simulink library "lib_TCML"  (R2015a)
settings: Solver=ode45  StartTime=0.0  StopTime=10.0  RelTol=1e-3
libraries: simulink x5
(part 4 of 7)

== system lib_TCML/Dynamic Tip Clearance/Case Deformation/Deformation1 ==
  Average Temperature(R) : Inport
  Memory : Memory  X0=mean(T0_Case_M)
  Memory3 : Memory  X0=Ri_Case_M
  Thermal Expansion 1D Elastic : Subsystem  mask(TSAT: Thermal Expansion Library Block){TempDependence_M=on, alpha_M=alpha_Case_M, T_data_M=Talpha_Case_Data_M, alpha_data_M=alpha_Case_Data_M, BN_M=double(gcb)}
      mask prompts: TempDependence_M "TempDependence_M - Temperature dependence of the thermal expansion coefficient (unchecked - constant, checked - temperature dependent)"; alpha_M "alpha_M - Constant thermal expansion coefficient"; T_data_M "T_data_M - Temperature array (nx1)"; alpha_data_M "alpha_data_M - Thermal expansion coefficient array (nx1)"; BN_M "Block Name"
      mask help:
      | This function calculates the length or radius of a structure that has expanded or contracted due to thermal expansion. The block accepts the previous/reference length (Lo), previous/reference temperature (To), and current temperature (Tf) as its inputs. The user has the option to specify a constant thermal expansion coefficient or to incorporate temperature dependence by providing data that correlates the thermal expansion coefficient with temperature.
      |
      | This block is capable of accepting various units but it is important that the units be consistent across all inputs and parameters. For details on this block, see the block help menu.
      mask init:
      | %set default parameters if they are not being used
      | if TempDependence_M == 0
      |     T_data_M = [0 5000];
      |     alpha_data_M = [10e-6 10e-6];
      | elseif TempDependence_M == 1
      |     alpha_M = 10e-6;
      | end
      mask Help: web(which('Deformation_TSAT_ThermExp1DElastic.html'),'-helpbrowser')
      mask Callback TempDependence_M:
      | MSK_SEC_Enables_TSAT('TempDependence_M',2,'dis')
      | MSK_SEC_Enables_TSAT('TempDependence_M',[3 4],'en')
  Case Radius (ft) : Outport
  wires:
  Thermal Expansion 1D Elastic/1(Current Length [L]) -> Memory3/1, Case Radius (ft)/1
  Average Temperature(R)/1 -> Memory/1, Thermal Expansion 1D Elastic/3(Current Temperature [Tf])
  Memory/1 -> Thermal Expansion 1D Elastic/2(Previous/Reference Temperature [To])
  Memory3/1 -> Thermal Expansion 1D Elastic/1(Previous/Reference Length [Lo])

== system lib_TCML/Dynamic Tip Clearance/Case Deformation/Thermal Properties ==
  Temperature [T] : Inport
  Density (Abradable Material) : Constant  Value=rho_Case_M * ones(1,n_Case_M)  SampleTime=dt_Case_M
  Heat Capacity vs. Temperature (Abradable Material) : Lookup_n-D  NumberOfTableDimensions=1  BreakpointsForDimension1=TCp_Case_Data_M  Table=Cp_Case_Data_M  InternalRulePriority=Speed  RndMeth=Simplest  InputSameDT=on
  Is k of temperature dependent : Constant  Value=k_TempDependence_Case_M  SampleTime=dt_Case_M
  Is k of temperature dependent1 : Constant  Value=Cp_TempDependence_Case_M  SampleTime=dt_Case_M
  Switch1 : Switch  Criteria=u2 > Threshold
  Switch2 : Switch  Criteria=u2 > Threshold
  Thermal Conductivity (Abradable Material) : Constant  Value=k_Case_M * ones(1,n_Case_M)  SampleTime=dt_Case_M
  Thermal Conductivity (Abradable Material)1 : Constant  Value=Cp_Case_M * ones(1,n_Case_M)  SampleTime=dt_Case_M
  Thermal Conductivity vs. Temperature (Abradable Material) : Lookup_n-D  NumberOfTableDimensions=1  BreakpointsForDimension1=Tk_Case_Data_M  Table=k_Case_Data_M  InternalRulePriority=Speed  RndMeth=Simplest  InputSameDT=on
  Thermal Conductivity [k] : Outport
  Heat Capacity [Cp] : Outport  Port=2
  Density [rho] : Outport  Port=3
  wires:
  Switch1/1 -> Heat Capacity [Cp]/1
  Is k of temperature dependent1/1 -> Switch1/2
  Thermal Conductivity (Abradable Material)1/1 -> Switch1/3
  Is k of temperature dependent/1 -> Switch2/2
  Thermal Conductivity (Abradable Material)/1 -> Switch2/3
  Thermal Conductivity vs. Temperature (Abradable Material)/1 -> Switch2/1
  Switch2/1 -> Thermal Conductivity [k]/1
  Density (Abradable Material)/1 -> Density [rho]/1
  Temperature [T]/1 -> Thermal Conductivity vs. Temperature (Abradable Material)/1, Heat Capacity vs. Temperature (Abradable Material)/1
  Heat Capacity vs. Temperature (Abradable Material)/1 -> Switch1/1

== system lib_TCML/Dynamic Tip Clearance/Case Deformation/While Iterator Subsystem ==
  Tin (R)1 : Inport
  hin (Btu/(sec-ft^2-R))1 : Inport  Port=2
  Tout (R)1 : Inport  Port=3
  hout (Btu/(sec-ft^2-R))1 : Inport  Port=4
  Abs2 : Abs
  Add2 : Sum  Inputs=-+
  Compare To Constant2 : simulink/Logic and Bit Operations/Compare To Constant  relop=>=  const=0.1  OutDataTypeStr=boolean
  Is k of temperature dependent1 : Constant  Value=k_TempDependence_Case_M  SampleTime=-1
  MATLAB Function1 : MATLAB Function  TreatAsAtomicUnit=on
  Memory5 : Memory  X0=mean(T0_Case_M)  InheritSampleTime=on
  Memory6 : Memory  X0=mean(T0_Case_M)  InheritSampleTime=on
  Switch : Switch  Criteria=u2 > Threshold
  Thermal Conductivity (Abradable Material)1 : Constant  Value=k_Case_M  SampleTime=-1
  Thermal Conductivity vs. Temperature : Lookup_n-D  NumberOfTableDimensions=1  BreakpointsForDimension1=Tk_Case_Data_M  Table=k_Case_Data_M  InternalRulePriority=Speed  RndMeth=Simplest  InputSameDT=on
  While Iterator : WhileIterator  MaxIters=1000  WhileBlockType=do-while
  Width of Rotor : Constant  Value=W_Case_M  SampleTime=-1
  Tavg (R) : Outport
  wires:
  Thermal Conductivity vs. Temperature/1 -> Switch/1
  Is k of temperature dependent1/1 -> Switch/2
  Thermal Conductivity (Abradable Material)1/1 -> Switch/3
  Compare To Constant2/1 -> While Iterator/1
  Abs2/1 -> Compare To Constant2/1
  Add2/1 -> Abs2/1
  Memory5/1 -> Add2/1
  Memory6/1 -> Thermal Conductivity vs. Temperature/1
  MATLAB Function1/1(Tavg) -> Memory5/1, Memory6/1, Add2/2, Tavg (R)/1
  Switch/1 -> MATLAB Function1/1(k)
  hout (Btu/(sec-ft^2-R))1/1 -> MATLAB Function1/6(hout)
  Tout (R)1/1 -> MATLAB Function1/5(Tout)
  hin (Btu/(sec-ft^2-R))1/1 -> MATLAB Function1/4(hin)
  Tin (R)1/1 -> MATLAB Function1/3(Tin)
  Width of Rotor/1 -> MATLAB Function1/2(W)

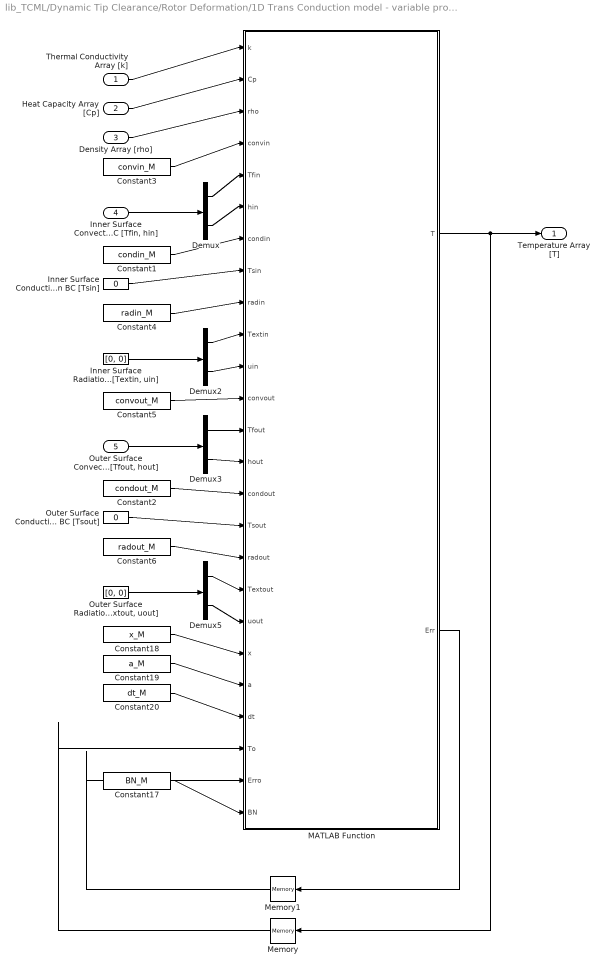
== system lib_TCML/Dynamic Tip Clearance/Rotor Deformation/1D Trans Conduction model - variable props & general BCs ==
  Thermal Conductivity Array [k] : Inport
  Heat Capacity Array [Cp] : Inport  Port=2
  Density Array [rho] : Inport  Port=3
  "Inner Surface Convection BC [Tfin, hin]" : Inport  Port=4
  "Outer Surface Convection BC [Tfout, hout]" : Inport  Port=5
  Constant1 : Constant  Value=condin_M
  Constant17 : Constant  Value=BN_M
  Constant18 : Constant  Value=x_M
  Constant19 : Constant  Value=a_M
  Constant2 : Constant  Value=condout_M
  Constant20 : Constant  Value=dt_M
  Constant3 : Constant  Value=convin_M
  Constant4 : Constant  Value=radin_M
  Constant5 : Constant  Value=convout_M
  Constant6 : Constant  Value=radout_M
  Demux{,2..3,5} (4 alike) : Demux  Outputs=[1 1]
  Inner Surface Conduction BC [Tsin] : Constant  Value=0
  "Inner Surface Radiation BC [Textin, uin]" : Constant  Value=[0, 0]
  MATLAB Function : MATLAB Function  TreatAsAtomicUnit=on  SystemSampleTime=dt_M
  Memory : Memory  X0=T0_M  InheritSampleTime=on
  Memory1 : Memory  X0=zeros(1,37)  InheritSampleTime=on
  Outer Surface Conduction BC [Tsout] : Constant  Value=0
  "Outer Surface Radiation BC [Textout, uout]" : Constant  Value=[0, 0]
  Temperature Array [T] : Outport
  wires:
  "Outer Surface Radiation BC [Textout, uout]"/1 -> Demux5/1
  Demux5/2 -> MATLAB Function/19(uout)
  Demux5/1 -> MATLAB Function/18(Textout)
  Outer Surface Conduction BC [Tsout]/1 -> MATLAB Function/16(Tsout)
  Demux3/2 -> MATLAB Function/14(hout)
  Demux3/1 -> MATLAB Function/13(Tfout)
  "Outer Surface Convection BC [Tfout, hout]"/1 -> Demux3/1
  Demux2/2 -> MATLAB Function/11(uin)
  Demux2/1 -> MATLAB Function/10(Textin)
  "Inner Surface Radiation BC [Textin, uin]"/1 -> Demux2/1
  Inner Surface Conduction BC [Tsin]/1 -> MATLAB Function/8(Tsin)
  Demux/2 -> MATLAB Function/6(hin)
  Demux/1 -> MATLAB Function/5(Tfin)
  "Inner Surface Convection BC [Tfin, hin]"/1 -> Demux/1
  Constant6/1 -> MATLAB Function/17(radout)
  Constant5/1 -> MATLAB Function/12(convout)
  Constant4/1 -> MATLAB Function/9(radin)
  Constant3/1 -> MATLAB Function/4(convin)
  Constant2/1 -> MATLAB Function/15(condout)
  Constant1/1 -> MATLAB Function/7(condin)
  MATLAB Function/2(Err) -> Memory1/1
  Memory/1 -> MATLAB Function/23(To)
  MATLAB Function/1(T) -> Temperature Array [T]/1, Memory/1
  Constant20/1 -> MATLAB Function/22(dt)
  Constant19/1 -> MATLAB Function/21(a)
  Constant18/1 -> MATLAB Function/20(x)
  Density Array [rho]/1 -> MATLAB Function/3(rho)
  Heat Capacity Array [Cp]/1 -> MATLAB Function/2(Cp)
  Thermal Conductivity Array [k]/1 -> MATLAB Function/1(k)
  Memory1/1 -> MATLAB Function/24(Erro)
  Constant17/1 -> MATLAB Function/25(BN)

== system lib_TCML/Dynamic Tip Clearance/Rotor Deformation/Convective Heat Transfer Coefficient on Back Surface ==
  Mass Flow Rate [W] : Inport
  Fluid Temperature [T] : Inport  Port=2
  2-D Lookup Table : Lookup_n-D  BreakpointsForDimension1=Wc_Rotor_Back_Data_M  BreakpointsForDimension2=Tc_Rotor_Back_Data_M  Table=h_Rotor_Back_Data_M  InternalRulePriority=Speed  RndMeth=Simplest  InputSameDT=on
  Constant : Constant  Value=0.8  SampleTime=dt_Rotor_M
  Constant1 : Constant  Value=0.23  SampleTime=dt_Rotor_M
  Convective Heat Transfer Coefficient : Constant  Value=h_Rotor_Back_M  SampleTime=dt_Rotor_M
  Gain : Gain  Gain=hcoeff_Rotor_Back_M
  Gain1 : Gain  Gain=1/Wdes_Rotor_Back_M
  Gain2 : Gain  Gain=1/Tdes_Rotor_Back_M
  Math Function : Math  Operator=pow  SaturateOnIntegerOverflow=on
  Math Function1 : Math  Operator=pow  SaturateOnIntegerOverflow=on
  Multiport Switch : MultiPortSwitch
  Product : Product
  Which Convective Heat Transfer Coefficient Model? : Constant  Value=ConvHeatXCoeffMdl_Rotor_Back_I  SampleTime=dt_Rotor_M
  Convective Heat Transfer Coefficient [h] : Outport
  wires:
  Multiport Switch/1 -> Convective Heat Transfer Coefficient [h]/1
  2-D Lookup Table/1 -> Multiport Switch/4
  Constant/1 -> Math Function/2
  Which Convective Heat Transfer Coefficient Model?/1 -> Multiport Switch/1
  Gain/1 -> Multiport Switch/3
  Mass Flow Rate [W]/1 -> Gain1/1
  Convective Heat Transfer Coefficient/1 -> Multiport Switch/2
  Gain1/1 -> 2-D Lookup Table/2, Math Function/1
  Constant1/1 -> Math Function1/2
  Fluid Temperature [T]/1 -> Gain2/1
  Gain2/1 -> 2-D Lookup Table/1, Math Function1/1
  Math Function/1 -> Product/1
  Math Function1/1 -> Product/2
  Product/1 -> Gain/1

== system lib_TCML/Dynamic Tip Clearance/Rotor Deformation/Convective Heat Transfer Coefficient on Front Surface ==
  Mass Flow Rate [W] : Inport
  Fluid Temperature [T] : Inport  Port=2
  2-D Lookup Table : Lookup_n-D  BreakpointsForDimension1=Wc_Rotor_Front_Data_M  BreakpointsForDimension2=Tc_Rotor_Front_Data_M  Table=h_Rotor_Front_Data_M  InternalRulePriority=Speed  RndMeth=Simplest  InputSameDT=on
  Constant : Constant  Value=0.8  SampleTime=dt_Rotor_M
  Constant1 : Constant  Value=0.23  SampleTime=dt_Rotor_M
  Convective Heat Transfer Coefficient : Constant  Value=h_Rotor_Front_M  SampleTime=dt_Rotor_M
  Gain : Gain  Gain=hcoeff_Rotor_Front_M
  Gain1 : Gain  Gain=1/Wdes_Rotor_Front_M
  Gain2 : Gain  Gain=1/Tdes_Rotor_Front_M
  Math Function : Math  Operator=pow  SaturateOnIntegerOverflow=on
  Math Function1 : Math  Operator=pow  SaturateOnIntegerOverflow=on
  Multiport Switch : MultiPortSwitch
  Product : Product
  Which Convective Heat Transfer Coefficient Model? : Constant  Value=ConvHeatXCoeffMdl_Rotor_Front_I  SampleTime=dt_Rotor_M
  Convective Heat Transfer Coefficient [h] : Outport
  wires:
  Product/1 -> Gain/1
  Math Function1/1 -> Product/2
  Math Function/1 -> Product/1
  Gain2/1 -> Math Function1/1, 2-D Lookup Table/1
  Fluid Temperature [T]/1 -> Gain2/1
  Constant1/1 -> Math Function1/2
  Gain1/1 -> Math Function/1, 2-D Lookup Table/2
  Convective Heat Transfer Coefficient/1 -> Multiport Switch/2
  Mass Flow Rate [W]/1 -> Gain1/1
  Gain/1 -> Multiport Switch/3
  Which Convective Heat Transfer Coefficient Model?/1 -> Multiport Switch/1
  Constant/1 -> Math Function/2
  2-D Lookup Table/1 -> Multiport Switch/4
  Multiport Switch/1 -> Convective Heat Transfer Coefficient [h]/1

== system lib_TCML/Dynamic Tip Clearance/Rotor Deformation/Deformation ==
  Average Temperature (R) : Inport
  Shaft Speed (rpm) : Inport  Port=2
  Deformation Due To Centrifugal Forces : Subsystem
  Deformation Due To Thermal Expansion : Subsystem
  Subtract : Sum
  Rotor Outer Radius (ft) : Outport
  Unstrained Rotor Outer Radius (ft) : Outport  Port=2
  wires:
  Average Temperature (R)/1 -> Deformation Due To Centrifugal Forces/2(Average Temperature), Deformation Due To Thermal Expansion/1(Average Rotor Temperature)
  Subtract/1 -> Rotor Outer Radius (ft)/1
  Shaft Speed (rpm)/1 -> Deformation Due To Centrifugal Forces/1(Shaft Speed [N] (rpm))
  Deformation Due To Centrifugal Forces/1(Rotor Radius) -> Subtract/1
  Deformation Due To Thermal Expansion/1(Rotor Radius after Thermal Expansion) -> Unstrained Rotor Outer Radius (ft)/1, Subtract/2, Deformation Due To Centrifugal Forces/3(Rotor Radius After Thermal Expansion)

== system lib_TCML/Dynamic Tip Clearance/Rotor Deformation/Deformation1 ==
  Average Temperature (R) : Inport
  Shaft Speed (rpm) : Inport  Port=2
  Deformation Due To Centrifugal Forces : Subsystem
  Deformation Due To Thermal Expansion : Subsystem
  Subtract : Sum
  Rotor Outer Radius (ft) : Outport
  wires:
  Deformation Due To Thermal Expansion/1(Rotor Radius after Thermal Expansion) -> Deformation Due To Centrifugal Forces/3(Rotor Radius After Thermal Expansion), Subtract/2
  Deformation Due To Centrifugal Forces/1(Rotor Radius) -> Subtract/1
  Shaft Speed (rpm)/1 -> Deformation Due To Centrifugal Forces/1(Shaft Speed [N] (rpm))
  Subtract/1 -> Rotor Outer Radius (ft)/1
  Average Temperature (R)/1 -> Deformation Due To Thermal Expansion/1(Average Rotor Temperature), Deformation Due To Centrifugal Forces/2(Average Temperature)

== system lib_TCML/Dynamic Tip Clearance/Rotor Deformation/Thermal Properties ==
  Temperature [T] : Inport
  Density (Super Alloy) : Constant  Value=rho_Rotor_M * ones(1,n_Rotor_M)  SampleTime=dt_Rotor_M
  Heat Capacity vs. Temperature : Lookup_n-D  NumberOfTableDimensions=1  BreakpointsForDimension1=TCp_Rotor_Data_M  Table=Cp_Rotor_Data_M  InternalRulePriority=Speed  RndMeth=Simplest  InputSameDT=on
  Is k of temperature dependent : Constant  Value=k_TempDependence_Rotor_M  SampleTime=dt_Rotor_M
  Is k of temperature dependent1 : Constant  Value=Cp_TempDependence_Rotor_M  SampleTime=dt_Rotor_M
  Switch : Switch  Criteria=u2 > Threshold
  Switch1 : Switch  Criteria=u2 > Threshold
  Thermal Conductivity (Abradable Material) : Constant  Value=k_Rotor_M * ones(1,n_Rotor_M)  SampleTime=dt_Rotor_M
  Thermal Conductivity (Super Alloy)1 : Constant  Value=Cp_Rotor_M * ones(1,n_Rotor_M)  SampleTime=dt_Rotor_M
  Thermal Conductivity vs. Temperature : Lookup_n-D  NumberOfTableDimensions=1  BreakpointsForDimension1=Tk_Rotor_Data_M  Table=k_Rotor_Data_M  InternalRulePriority=Speed  RndMeth=Simplest  InputSameDT=on
  Thermal Conductivity [k] : Outport
  Heat Capacity [Cp] : Outport  Port=2
  Density [rho] : Outport  Port=3
  wires:
  Temperature [T]/1 -> Heat Capacity vs. Temperature/1, Thermal Conductivity vs. Temperature/1
  Thermal Conductivity (Super Alloy)1/1 -> Switch1/3
  Thermal Conductivity vs. Temperature/1 -> Switch/1
  Switch/1 -> Thermal Conductivity [k]/1
  Is k of temperature dependent/1 -> Switch/2
  Heat Capacity vs. Temperature/1 -> Switch1/1
  Switch1/1 -> Heat Capacity [Cp]/1
  Is k of temperature dependent1/1 -> Switch1/2
  Thermal Conductivity (Abradable Material)/1 -> Switch/3
  Density (Super Alloy)/1 -> Density [rho]/1

== system lib_TCML/Dynamic Tip Clearance/Rotor Deformation/While Iterator Subsystem ==
  Tin (R) : Inport
  hin (Btu/(sec-ft^2-R)) : Inport  Port=2
  Tout (R) : Inport  Port=3
  hout (Btu/(sec-ft^2-R)) : Inport  Port=4
  Abs : Abs
  Add : Sum  Inputs=-+
  Compare To Constant : simulink/Logic and Bit Operations/Compare To Constant  relop=>=  const=0.1  OutDataTypeStr=boolean
  Is k of temperature dependent : Constant  Value=k_TempDependence_Rotor_M  SampleTime=-1
  MATLAB Function1 : MATLAB Function  TreatAsAtomicUnit=on
  Memory1 : Memory  X0=mean(T0_Rotor_M)  InheritSampleTime=on
  Memory2 : Memory  X0=mean(T0_Rotor_M)  InheritSampleTime=on
  Switch : Switch  Criteria=u2 > Threshold
  Thermal Conductivity (Abradable Material) : Constant  Value=k_Rotor_M  SampleTime=-1
  Thermal Conductivity vs. Temperature : Lookup_n-D  NumberOfTableDimensions=1  BreakpointsForDimension1=Tk_Rotor_Data_M  Table=k_Rotor_Data_M  InternalRulePriority=Speed  RndMeth=Simplest  InputSameDT=on
  While Iterator : WhileIterator  MaxIters=1000  WhileBlockType=do-while
  Width of Rotor : Constant  Value=W_Rotor_M  SampleTime=-1
  Tavg (R) : Outport
  wires:
  Thermal Conductivity vs. Temperature/1 -> Switch/1
  Is k of temperature dependent/1 -> Switch/2
  Thermal Conductivity (Abradable Material)/1 -> Switch/3
  Compare To Constant/1 -> While Iterator/1
  Abs/1 -> Compare To Constant/1
  Add/1 -> Abs/1
  Memory1/1 -> Add/1
  Memory2/1 -> Thermal Conductivity vs. Temperature/1
  MATLAB Function1/1(Tavg) -> Memory1/1, Memory2/1, Add/2, Tavg (R)/1
  Switch/1 -> MATLAB Function1/1(k)
  hout (Btu/(sec-ft^2-R))/1 -> MATLAB Function1/6(hout)
  Tout (R)/1 -> MATLAB Function1/5(Tout)
  hin (Btu/(sec-ft^2-R))/1 -> MATLAB Function1/4(hin)
  Tin (R)/1 -> MATLAB Function1/3(Tin)
  Width of Rotor/1 -> MATLAB Function1/2(W)

== system lib_TCML/Steady-State Tip Clearance/Blade Deformation/Deformation ==
  Average Temperature : Inport
  Shaft Speed [N] (rpm) : Inport  Port=2
  Rotor Outer Radius : Inport  Port=3
  Deformation Due To Centrifugal Forces : Subsystem
  Deformation Due To Thermal Expansion : Subsystem
  Subtract : Sum
  Blade Length : Outport
  Unstrained Blade Length : Outport  Port=2
  wires:
  Average Temperature/1 -> Deformation Due To Thermal Expansion/1(Average Rotor Temperature), Deformation Due To Centrifugal Forces/2(Average Temperature)
  Subtract/1 -> Blade Length/1
  Shaft Speed [N] (rpm)/1 -> Deformation Due To Centrifugal Forces/1(Shaft Speed [N] (rpm))
  Deformation Due To Centrifugal Forces/1(Blade Length) -> Subtract/1
  Deformation Due To Thermal Expansion/1(Blade Length after Thermal Expansion) -> Subtract/2, Unstrained Blade Length/1, Deformation Due To Centrifugal Forces/3(Blade Length After Thermal Expansion)
  Rotor Outer Radius/1 -> Deformation Due To Centrifugal Forces/4(Rotor Outer Radius)

== system lib_TCML/Steady-State Tip Clearance/Blade Deformation/Lumped Mass Heat Transfer Model ==
  Temperature of Core Flow [Tcore] : Inport
  Temperature of Cooling Flow [Tcool] : Inport  Port=2
  Add1 : Sum  Inputs=-+
  Add3 : Sum
  Gain : Gain  Gain=eta_Blade_M
  Reference Temperature [Tref] : Outport
  wires:
  Temperature of Cooling Flow [Tcool]/1 -> Add1/2
  Temperature of Core Flow [Tcore]/1 -> Add3/1, Add1/1
  Add3/1 -> Reference Temperature [Tref]/1  "T ref"
  Gain/1 -> Add3/2
  Add1/1 -> Gain/1

== system lib_TCML/Steady-State Tip Clearance/Case Deformation/Convective Heat Transfer Coefficient on Inner Surface ==
  Mass Flow Rate [W] : Inport
  Fluid Temperature [T] : Inport  Port=2
  2-D Lookup Table : Lookup_n-D  BreakpointsForDimension1=Wc_Case_In_Data_M  BreakpointsForDimension2=Tc_Case_In_Data_M  Table=h_Case_In_Data_M  InternalRulePriority=Speed  RndMeth=Simplest  InputSameDT=on
  Constant : Constant  Value=0.8
  Constant1 : Constant  Value=0.23
  Convective Heat Transfer Coefficient : Constant  Value=h_Case_In_M
  Gain : Gain  Gain=hcoeff_Case_In_M
  Gain1 : Gain  Gain=1/Wdes_Case_In_M
  Gain2 : Gain  Gain=1/Tdes_Case_In_M
  Math Function : Math  Operator=pow  SaturateOnIntegerOverflow=on
  Math Function1 : Math  Operator=pow  SaturateOnIntegerOverflow=on
  Multiport Switch : MultiPortSwitch
  Product : Product
  Which Convective Heat Transfer Coefficient Model? : Constant  Value=ConvHeatXCoeffMdl_Case_In_I
  Convective Heat Transfer Coefficient [h] : Outport
  wires:
  Multiport Switch/1 -> Convective Heat Transfer Coefficient [h]/1
  2-D Lookup Table/1 -> Multiport Switch/4
  Constant/1 -> Math Function/2
  Which Convective Heat Transfer Coefficient Model?/1 -> Multiport Switch/1
  Gain/1 -> Multiport Switch/3
  Mass Flow Rate [W]/1 -> Gain1/1
  Convective Heat Transfer Coefficient/1 -> Multiport Switch/2
  Gain1/1 -> 2-D Lookup Table/2, Math Function/1
  Constant1/1 -> Math Function1/2
  Fluid Temperature [T]/1 -> Gain2/1
  Gain2/1 -> 2-D Lookup Table/1, Math Function1/1
  Math Function/1 -> Product/1
  Math Function1/1 -> Product/2
  Product/1 -> Gain/1

== system lib_TCML/Steady-State Tip Clearance/Case Deformation/Convective Heat Transfer Coefficient on Outer Surface ==
  Mass Flow Rate [W] : Inport
  Fluid Temperature [T] : Inport  Port=2
  2-D Lookup Table : Lookup_n-D  BreakpointsForDimension1=Wc_Case_Out_Data_M  BreakpointsForDimension2=Tc_Case_Out_Data_M  Table=h_Case_Out_Data_M  InternalRulePriority=Speed  RndMeth=Simplest  InputSameDT=on
  Constant : Constant  Value=0.8
  Constant1 : Constant  Value=0.23
  Convective Heat Transfer Coefficient : Constant  Value=h_Case_Out_M
  Gain : Gain  Gain=hcoeff_Case_Out_M
  Gain1 : Gain  Gain=1/Wdes_Case_Out_M
  Gain2 : Gain  Gain=1/Tdes_Case_Out_M
  Math Function : Math  Operator=pow  SaturateOnIntegerOverflow=on
  Math Function1 : Math  Operator=pow  SaturateOnIntegerOverflow=on
  Multiport Switch : MultiPortSwitch
  Product : Product
  Which Convective Heat Transfer Coefficient Model? : Constant  Value=ConvHeatXCoeffMdl_Case_Out_I
  Convective Heat Transfer Coefficient [h] : Outport
  wires:
  Product/1 -> Gain/1
  Math Function1/1 -> Product/2
  Math Function/1 -> Product/1
  Gain2/1 -> Math Function1/1, 2-D Lookup Table/1
  Fluid Temperature [T]/1 -> Gain2/1
  Constant1/1 -> Math Function1/2
  Gain1/1 -> Math Function/1, 2-D Lookup Table/2
  Convective Heat Transfer Coefficient/1 -> Multiport Switch/2
  Mass Flow Rate [W]/1 -> Gain1/1
  Gain/1 -> Multiport Switch/3
  Which Convective Heat Transfer Coefficient Model?/1 -> Multiport Switch/1
  Constant/1 -> Math Function/2
  2-D Lookup Table/1 -> Multiport Switch/4
  Multiport Switch/1 -> Convective Heat Transfer Coefficient [h]/1

== system lib_TCML/Steady-State Tip Clearance/Case Deformation/Convective Heat Transfer Coefficient on Outer Surface1 ==
  Mass Flow Rate [W] : Inport
  Fluid Temperature [T] : Inport  Port=2
  2-D Lookup Table : Lookup_n-D  BreakpointsForDimension1=Wc_Case_Out_Data_M  BreakpointsForDimension2=Tc_Case_Out_Data_M  Table=h_Case_Out_Data_M  InternalRulePriority=Speed  RndMeth=Simplest  InputSameDT=on
  Constant : Constant  Value=0.8
  Constant1 : Constant  Value=0.23
  Convective Heat Transfer Coefficient : Constant  Value=h_Case_Out_M
  Gain : Gain  Gain=hcoeff_Case_Out_M
  Gain1 : Gain  Gain=1/Wdes_Case_Out_M
  Gain2 : Gain  Gain=1/Tdes_Case_Out_M
  Math Function : Math  Operator=pow  SaturateOnIntegerOverflow=on
  Math Function1 : Math  Operator=pow  SaturateOnIntegerOverflow=on
  Multiport Switch : MultiPortSwitch
  Product : Product
  Which Convective Heat Transfer Coefficient Model? : Constant  Value=ConvHeatXCoeffMdl_Case_Out_I
  Convective Heat Transfer Coefficient [h] : Outport
  wires:
  Multiport Switch/1 -> Convective Heat Transfer Coefficient [h]/1
  2-D Lookup Table/1 -> Multiport Switch/4
  Constant/1 -> Math Function/2
  Which Convective Heat Transfer Coefficient Model?/1 -> Multiport Switch/1
  Gain/1 -> Multiport Switch/3
  Mass Flow Rate [W]/1 -> Gain1/1
  Convective Heat Transfer Coefficient/1 -> Multiport Switch/2
  Gain1/1 -> 2-D Lookup Table/2, Math Function/1
  Constant1/1 -> Math Function1/2
  Fluid Temperature [T]/1 -> Gain2/1
  Gain2/1 -> 2-D Lookup Table/1, Math Function1/1
  Math Function/1 -> Product/1
  Math Function1/1 -> Product/2
  Product/1 -> Gain/1

== system lib_TCML/Steady-State Tip Clearance/Case Deformation/Deformation ==
  Average Temperature(R) : Inport
  Memory : Memory  X0=mean(T0_Case_M)
  Memory3 : Memory  X0=Ri_Case_M
  Thermal Expansion 1D Elastic : Subsystem  mask(TSAT: Thermal Expansion Library Block){TempDependence_M=on, alpha_M=alpha_Case_M, T_data_M=Talpha_Case_Data_M, alpha_data_M=alpha_Case_Data_M, BN_M=double(gcb)}
      mask prompts: TempDependence_M "TempDependence_M - Temperature dependence of the thermal expansion coefficient (unchecked - constant, checked - temperature dependent)"; alpha_M "alpha_M - Constant thermal expansion coefficient"; T_data_M "T_data_M - Temperature array (nx1)"; alpha_data_M "alpha_data_M - Thermal expansion coefficient array (nx1)"; BN_M "Block Name"
      mask help:
      | This function calculates the length or radius of a structure that has expanded or contracted due to thermal expansion. The block accepts the previous/reference length (Lo), previous/reference temperature (To), and current temperature (Tf) as its inputs. The user has the option to specify a constant thermal expansion coefficient or to incorporate temperature dependence by providing data that correlates the thermal expansion coefficient with temperature.
      |
      | This block is capable of accepting various units but it is important that the units be consistent across all inputs and parameters. For details on this block, see the block help menu.
      mask init:
      | %set default parameters if they are not being used
      | if TempDependence_M == 0
      |     T_data_M = [0 5000];
      |     alpha_data_M = [10e-6 10e-6];
      | elseif TempDependence_M == 1
      |     alpha_M = 10e-6;
      | end
      mask Help: web(which('Deformation_TSAT_ThermExp1DElastic.html'),'-helpbrowser')
      mask Callback TempDependence_M:
      | MSK_SEC_Enables_TSAT('TempDependence_M',2,'dis')
      | MSK_SEC_Enables_TSAT('TempDependence_M',[3 4],'en')
  Case Radius (ft) : Outport
  wires:
  Thermal Expansion 1D Elastic/1(Current Length [L]) -> Memory3/1, Case Radius (ft)/1
  Average Temperature(R)/1 -> Memory/1, Thermal Expansion 1D Elastic/3(Current Temperature [Tf])
  Memory/1 -> Thermal Expansion 1D Elastic/2(Previous/Reference Temperature [To])
  Memory3/1 -> Thermal Expansion 1D Elastic/1(Previous/Reference Length [Lo])

== system lib_TCML/Steady-State Tip Clearance/Case Deformation/Deformation1 ==
  Average Temperature(R) : Inport
  Memory : Memory  X0=mean(T0_Case_M)
  Memory3 : Memory  X0=Ri_Case_M
  Thermal Expansion 1D Elastic : Subsystem  mask(TSAT: Thermal Expansion Library Block){TempDependence_M=on, alpha_M=alpha_Case_M, T_data_M=Talpha_Case_Data_M, alpha_data_M=alpha_Case_Data_M, BN_M=double(gcb)}
      mask prompts: TempDependence_M "TempDependence_M - Temperature dependence of the thermal expansion coefficient (unchecked - constant, checked - temperature dependent)"; alpha_M "alpha_M - Constant thermal expansion coefficient"; T_data_M "T_data_M - Temperature array (nx1)"; alpha_data_M "alpha_data_M - Thermal expansion coefficient array (nx1)"; BN_M "Block Name"
      mask help:
      | This function calculates the length or radius of a structure that has expanded or contracted due to thermal expansion. The block accepts the previous/reference length (Lo), previous/reference temperature (To), and current temperature (Tf) as its inputs. The user has the option to specify a constant thermal expansion coefficient or to incorporate temperature dependence by providing data that correlates the thermal expansion coefficient with temperature.
      |
      | This block is capable of accepting various units but it is important that the units be consistent across all inputs and parameters. For details on this block, see the block help menu.
      mask init:
      | %set default parameters if they are not being used
      | if TempDependence_M == 0
      |     T_data_M = [0 5000];
      |     alpha_data_M = [10e-6 10e-6];
      | elseif TempDependence_M == 1
      |     alpha_M = 10e-6;
      | end
      mask Help: web(which('Deformation_TSAT_ThermExp1DElastic.html'),'-helpbrowser')
      mask Callback TempDependence_M:
      | MSK_SEC_Enables_TSAT('TempDependence_M',2,'dis')
      | MSK_SEC_Enables_TSAT('TempDependence_M',[3 4],'en')
  Case Radius (ft) : Outport
  wires:
  Memory3/1 -> Thermal Expansion 1D Elastic/1(Previous/Reference Length [Lo])
  Memory/1 -> Thermal Expansion 1D Elastic/2(Previous/Reference Temperature [To])
  Average Temperature(R)/1 -> Thermal Expansion 1D Elastic/3(Current Temperature [Tf]), Memory/1
  Thermal Expansion 1D Elastic/1(Current Length [L]) -> Case Radius (ft)/1, Memory3/1

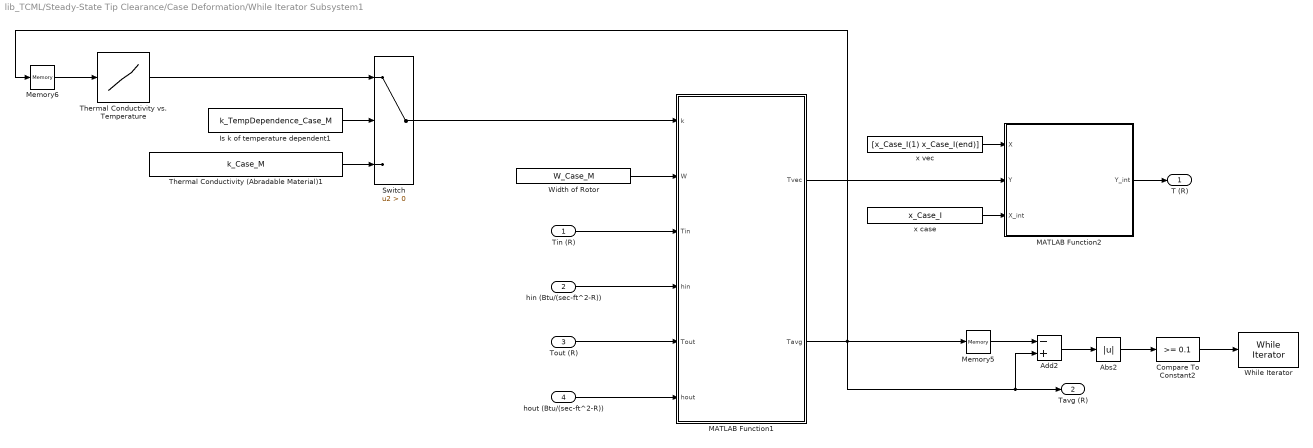
== system lib_TCML/Steady-State Tip Clearance/Case Deformation/While Iterator Subsystem1 ==
  Tin (R) : Inport
  hin (Btu/(sec-ft^2-R)) : Inport  Port=2
  Tout (R) : Inport  Port=3
  hout (Btu/(sec-ft^2-R)) : Inport  Port=4
  Abs2 : Abs
  Add2 : Sum  Inputs=-+
  Compare To Constant2 : simulink/Logic and Bit Operations/Compare To Constant  relop=>=  const=0.1  OutDataTypeStr=boolean
  Is k of temperature dependent1 : Constant  Value=k_TempDependence_Case_M  SampleTime=-1
  MATLAB Function1 : MATLAB Function  TreatAsAtomicUnit=on
  MATLAB Function2 : MATLAB Function  TreatAsAtomicUnit=on
  Memory5 : Memory  X0=mean(T0_Case_M)  InheritSampleTime=on
  Memory6 : Memory  X0=mean(T0_Case_M)  InheritSampleTime=on
  Switch : Switch  Criteria=u2 > Threshold
  Thermal Conductivity (Abradable Material)1 : Constant  Value=k_Case_M  SampleTime=-1
  Thermal Conductivity vs. Temperature : Lookup_n-D  NumberOfTableDimensions=1  BreakpointsForDimension1=Tk_Case_Data_M  Table=k_Case_Data_M  InternalRulePriority=Speed  RndMeth=Simplest  InputSameDT=on
  While Iterator : WhileIterator  MaxIters=1000  WhileBlockType=do-while
  Width of Rotor : Constant  Value=W_Case_M  SampleTime=-1
  x case : Constant  Value=x_Case_I  VectorParams1D=off  SampleTime=-1
  x vec : Constant  Value=[x_Case_I(1) x_Case_I(end)]  VectorParams1D=off  SampleTime=-1
  T (R) : Outport
  Tavg (R) : Outport  Port=2
  wires:
  MATLAB Function2/1(Y_int) -> T (R)/1
  x vec/1 -> MATLAB Function2/1(X)
  MATLAB Function1/1(Tvec) -> MATLAB Function2/2(Y)
  x case/1 -> MATLAB Function2/3(X_int)
  Thermal Conductivity vs. Temperature/1 -> Switch/1
  Is k of temperature dependent1/1 -> Switch/2
  Thermal Conductivity (Abradable Material)1/1 -> Switch/3
  Compare To Constant2/1 -> While Iterator/1
  Abs2/1 -> Compare To Constant2/1
  Add2/1 -> Abs2/1
  Memory5/1 -> Add2/1
  Memory6/1 -> Thermal Conductivity vs. Temperature/1
  MATLAB Function1/2(Tavg) -> Add2/2, Tavg (R)/1, Memory5/1, Memory6/1
  Switch/1 -> MATLAB Function1/1(k)
  hout (Btu/(sec-ft^2-R))/1 -> MATLAB Function1/6(hout)
  Tout (R)/1 -> MATLAB Function1/5(Tout)
  hin (Btu/(sec-ft^2-R))/1 -> MATLAB Function1/4(hin)
  Tin (R)/1 -> MATLAB Function1/3(Tin)
  Width of Rotor/1 -> MATLAB Function1/2(W)

== system lib_TCML/Steady-State Tip Clearance/Case Deformation/While Iterator Subsystem2 ==
  Tin (R) : Inport
  hin (Btu/(sec-ft^2-R)) : Inport  Port=2
  Tout (R) : Inport  Port=3
  hout (Btu/(sec-ft^2-R)) : Inport  Port=4
  Abs2 : Abs
  Add2 : Sum  Inputs=-+
  Compare To Constant2 : simulink/Logic and Bit Operations/Compare To Constant  relop=>=  const=0.1  OutDataTypeStr=boolean
  Is k of temperature dependent1 : Constant  Value=k_TempDependence_Case_M  SampleTime=-1
  MATLAB Function1 : MATLAB Function  TreatAsAtomicUnit=on
  MATLAB Function2 : MATLAB Function  TreatAsAtomicUnit=on
  Memory5 : Memory  X0=mean(T0_Case_M)  InheritSampleTime=on
  Memory6 : Memory  X0=mean(T0_Case_M)  InheritSampleTime=on
  Switch : Switch  Criteria=u2 > Threshold
  Thermal Conductivity (Abradable Material)1 : Constant  Value=k_Case_M  SampleTime=-1
  Thermal Conductivity vs. Temperature : Lookup_n-D  NumberOfTableDimensions=1  BreakpointsForDimension1=Tk_Case_Data_M  Table=k_Case_Data_M  InternalRulePriority=Speed  RndMeth=Simplest  InputSameDT=on
  While Iterator : WhileIterator  MaxIters=1000  WhileBlockType=do-while
  Width of Rotor : Constant  Value=W_Case_M  SampleTime=-1
  x case : Constant  Value=x_Case_I  VectorParams1D=off  SampleTime=-1
  x vec : Constant  Value=[x_Case_I(1) x_Case_I(end)]  VectorParams1D=off  SampleTime=-1
  T (R) : Outport
  Tavg (R) : Outport  Port=2
  wires:
  Width of Rotor/1 -> MATLAB Function1/2(W)
  Tin (R)/1 -> MATLAB Function1/3(Tin)
  hin (Btu/(sec-ft^2-R))/1 -> MATLAB Function1/4(hin)
  Tout (R)/1 -> MATLAB Function1/5(Tout)
  hout (Btu/(sec-ft^2-R))/1 -> MATLAB Function1/6(hout)
  Switch/1 -> MATLAB Function1/1(k)
  MATLAB Function1/2(Tavg) -> Memory6/1, Memory5/1, Tavg (R)/1, Add2/2
  Memory6/1 -> Thermal Conductivity vs. Temperature/1
  Memory5/1 -> Add2/1
  Add2/1 -> Abs2/1
  Abs2/1 -> Compare To Constant2/1
  Compare To Constant2/1 -> While Iterator/1
  Thermal Conductivity (Abradable Material)1/1 -> Switch/3
  Is k of temperature dependent1/1 -> Switch/2
  Thermal Conductivity vs. Temperature/1 -> Switch/1
  x case/1 -> MATLAB Function2/3(X_int)
  MATLAB Function1/1(Tvec) -> MATLAB Function2/2(Y)
  x vec/1 -> MATLAB Function2/1(X)
  MATLAB Function2/1(Y_int) -> T (R)/1

== system lib_TCML/Steady-State Tip Clearance/Rotor Deformation/Convective Heat Transfer Coefficient on Back Surface ==
  Mass Flow Rate [W] : Inport
  Fluid Temperature [T] : Inport  Port=2
  2-D Lookup Table : Lookup_n-D  BreakpointsForDimension1=Wc_Rotor_Back_Data_M  BreakpointsForDimension2=Tc_Rotor_Back_Data_M  Table=h_Rotor_Back_Data_M  InternalRulePriority=Speed  RndMeth=Simplest  InputSameDT=on
  Constant : Constant  Value=0.8
  Constant1 : Constant  Value=0.23
  Convective Heat Transfer Coefficient : Constant  Value=h_Rotor_Back_M
  Gain : Gain  Gain=hcoeff_Rotor_Back_M
  Gain1 : Gain  Gain=1/Wdes_Rotor_Back_M
  Gain2 : Gain  Gain=1/Tdes_Rotor_Back_M
  Math Function : Math  Operator=pow  SaturateOnIntegerOverflow=on
  Math Function1 : Math  Operator=pow  SaturateOnIntegerOverflow=on
  Multiport Switch : MultiPortSwitch
  Product : Product
  Which Convective Heat Transfer Coefficient Model? : Constant  Value=ConvHeatXCoeffMdl_Rotor_Back_I
  Convective Heat Transfer Coefficient [h] : Outport
  wires:
  Product/1 -> Gain/1
  Math Function1/1 -> Product/2
  Math Function/1 -> Product/1
  Gain2/1 -> Math Function1/1, 2-D Lookup Table/1
  Fluid Temperature [T]/1 -> Gain2/1
  Constant1/1 -> Math Function1/2
  Gain1/1 -> Math Function/1, 2-D Lookup Table/2
  Convective Heat Transfer Coefficient/1 -> Multiport Switch/2
  Mass Flow Rate [W]/1 -> Gain1/1
  Gain/1 -> Multiport Switch/3
  Which Convective Heat Transfer Coefficient Model?/1 -> Multiport Switch/1
  Constant/1 -> Math Function/2
  2-D Lookup Table/1 -> Multiport Switch/4
  Multiport Switch/1 -> Convective Heat Transfer Coefficient [h]/1

== system lib_TCML/Steady-State Tip Clearance/Rotor Deformation/Convective Heat Transfer Coefficient on Front Surface ==
  Mass Flow Rate [W] : Inport
  Fluid Temperature [T] : Inport  Port=2
  2-D Lookup Table : Lookup_n-D  BreakpointsForDimension1=Wc_Rotor_Front_Data_M  BreakpointsForDimension2=Tc_Rotor_Front_Data_M  Table=h_Rotor_Front_Data_M  InternalRulePriority=Speed  RndMeth=Simplest  InputSameDT=on
  Constant : Constant  Value=0.8
  Constant1 : Constant  Value=0.23
  Convective Heat Transfer Coefficient : Constant  Value=h_Rotor_Front_M
  Gain : Gain  Gain=hcoeff_Rotor_Front_M
  Gain1 : Gain  Gain=1/Wdes_Rotor_Front_M
  Gain2 : Gain  Gain=1/Tdes_Rotor_Front_M
  Math Function : Math  Operator=pow  SaturateOnIntegerOverflow=on
  Math Function1 : Math  Operator=pow  SaturateOnIntegerOverflow=on
  Multiport Switch : MultiPortSwitch
  Product : Product
  Which Convective Heat Transfer Coefficient Model? : Constant  Value=ConvHeatXCoeffMdl_Rotor_Front_I
  Convective Heat Transfer Coefficient [h] : Outport
  wires:
  Multiport Switch/1 -> Convective Heat Transfer Coefficient [h]/1
  2-D Lookup Table/1 -> Multiport Switch/4
  Constant/1 -> Math Function/2
  Which Convective Heat Transfer Coefficient Model?/1 -> Multiport Switch/1
  Gain/1 -> Multiport Switch/3
  Mass Flow Rate [W]/1 -> Gain1/1
  Convective Heat Transfer Coefficient/1 -> Multiport Switch/2
  Gain1/1 -> 2-D Lookup Table/2, Math Function/1
  Constant1/1 -> Math Function1/2
  Fluid Temperature [T]/1 -> Gain2/1
  Gain2/1 -> 2-D Lookup Table/1, Math Function1/1
  Math Function/1 -> Product/1
  Math Function1/1 -> Product/2
  Product/1 -> Gain/1

== system lib_TCML/Steady-State Tip Clearance/Rotor Deformation/Deformation ==
  Average Temperature (R) : Inport
  Shaft Speed (rpm) : Inport  Port=2
  Deformation Due To Centrifugal Forces : Subsystem
  Deformation Due To Thermal Expansion : Subsystem
  Subtract : Sum
  Rotor Outer Radius (ft) : Outport
  Unstrained Rotor Outer Radius (ft) : Outport  Port=2
  wires:
  Average Temperature (R)/1 -> Deformation Due To Centrifugal Forces/2(Average Temperature), Deformation Due To Thermal Expansion/1(Average Rotor Temperature)
  Subtract/1 -> Rotor Outer Radius (ft)/1
  Shaft Speed (rpm)/1 -> Deformation Due To Centrifugal Forces/1(Shaft Speed [N] (rpm))
  Deformation Due To Centrifugal Forces/1(Rotor Radius) -> Subtract/1
  Deformation Due To Thermal Expansion/1(Rotor Radius after Thermal Expansion) -> Unstrained Rotor Outer Radius (ft)/1, Subtract/2, Deformation Due To Centrifugal Forces/3(Rotor Radius After Thermal Expansion)

== system lib_TCML/Steady-State Tip Clearance/Rotor Deformation/While Iterator Subsystem ==
  Tin (R) : Inport
  hin (Btu/(sec-ft^2-R)) : Inport  Port=2
  Tout (R) : Inport  Port=3
  hout (Btu/(sec-ft^2-R)) : Inport  Port=4
  Abs : Abs
  Add : Sum  Inputs=-+
  Compare To Constant : simulink/Logic and Bit Operations/Compare To Constant  relop=>=  const=0.001  OutDataTypeStr=boolean
  Is k of temperature dependent : Constant  Value=k_TempDependence_Rotor_M  SampleTime=-1
  MATLAB Function : MATLAB Function  TreatAsAtomicUnit=on
  MATLAB Function1 : MATLAB Function  TreatAsAtomicUnit=on
  Memory1 : Memory  X0=mean(T0_Rotor_M)  InheritSampleTime=on
  Memory2 : Memory  X0=mean(T0_Rotor_M)  InheritSampleTime=on
  Switch : Switch  Criteria=u2 > Threshold
  Thermal Conductivity (Abradable Material) : Constant  Value=k_Rotor_M  SampleTime=-1
  Thermal Conductivity vs. Temperature : Lookup_n-D  NumberOfTableDimensions=1  BreakpointsForDimension1=Tk_Rotor_Data_M  Table=k_Rotor_Data_M  InternalRulePriority=Speed  RndMeth=Simplest  InputSameDT=on
  While Iterator : WhileIterator  MaxIters=1000  WhileBlockType=do-while
  Width of Rotor : Constant  Value=W_Rotor_M  SampleTime=-1
  x rotor : Constant  Value=x_Rotor_I  SampleTime=-1
  T (R) : Outport
  Tavg (R) : Outport  Port=2
  wires:
  MATLAB Function1/1(Y_int) -> T (R)/1
  x rotor/1 -> MATLAB Function1/3(X_int)
  MATLAB Function/1(x) -> MATLAB Function1/1(X)
  MATLAB Function/2(T) -> MATLAB Function1/2(Y)
  Width of Rotor/1 -> MATLAB Function/2(W)
  Tin (R)/1 -> MATLAB Function/3(Tin)
  hin (Btu/(sec-ft^2-R))/1 -> MATLAB Function/4(hin)
  Tout (R)/1 -> MATLAB Function/5(Tout)
  hout (Btu/(sec-ft^2-R))/1 -> MATLAB Function/6(hout)
  Switch/1 -> MATLAB Function/1(k)
  MATLAB Function/3(Tavg) -> Memory2/1, Memory1/1, Tavg (R)/1, Add/2
  Memory2/1 -> Thermal Conductivity vs. Temperature/1
  Memory1/1 -> Add/1
  Add/1 -> Abs/1
  Abs/1 -> Compare To Constant/1
  Compare To Constant/1 -> While Iterator/1
  Thermal Conductivity (Abradable Material)/1 -> Switch/3
  Is k of temperature dependent/1 -> Switch/2
  Thermal Conductivity vs. Temperature/1 -> Switch/1

== system lib_TCML/Dynamic Tip Clearance/Blade Deformation/Deformation/Deformation Due To Centrifugal Forces ==
  Shaft Speed [N] (rpm) : Inport
  Average Temperature : Inport  Port=2
  Blade Length After Thermal Expansion : Inport  Port=3
  Rotor Outer Radius : Inport  Port=4
  Add : Sum
  Constant Young's Modulus : Constant  Value=E_Blade_M
  Density of Rotor : Constant  Value=rho_Blade_M
  Density of Rotor1 : Constant
  Divide : Product  Inputs=/*
  Divide1 : Product  Inputs=****
  Divide2 : Product  Inputs=**
  E Temperature Dependence? : Constant  Value=E_TempDependence_Blade_M
  Gain1 : Gain  Gain=2*pi/60
  Math Function : Math  Operator=square  SaturateOnIntegerOverflow=on
  Math Function2 : Math  Operator=square  SaturateOnIntegerOverflow=on
  Switch : Switch  Criteria=u2 > Threshold
  Young's Modulus vs. Temperature : Lookup_n-D  NumberOfTableDimensions=1  BreakpointsForDimension1=TE_Blade_Data_M  Table=E_Blade_Data_M  InternalRulePriority=Speed  RndMeth=Simplest  InputSameDT=on
  Blade Length : Outport
  wires:
  Young's Modulus vs. Temperature/1 -> Switch/1
  Density of Rotor1/1 -> Divide/2
  Constant Young's Modulus/1 -> Switch/3
  Divide/1 -> Divide1/1
  Switch/1 -> Divide/1
  Gain1/1 -> Math Function/1  "rad/sec"
  Density of Rotor/1 -> Divide1/3
  E Temperature Dependence?/1 -> Switch/2
  Math Function/1 -> Divide1/2
  Shaft Speed [N] (rpm)/1 -> Gain1/1
  Divide1/1 -> Blade Length/1
  Average Temperature/1 -> Young's Modulus vs. Temperature/1
  Blade Length After Thermal Expansion/1 -> Add/2, Math Function2/1
  Rotor Outer Radius/1 -> Add/1
  Add/1 -> Divide2/1
  Math Function2/1 -> Divide2/2
  Divide2/1 -> Divide1/4

== system lib_TCML/Dynamic Tip Clearance/Blade Deformation/Deformation/Deformation Due To Thermal Expansion ==
  Average Rotor Temperature : Inport
  Memory1 : Memory  X0=T0_Blade_M
  Memory2 : Memory  X0=L_Blade_M
  Thermal Expansion 1D Elastic : Subsystem  mask(TSAT: Thermal Expansion Library Block){TempDependence_M=on, alpha_M=alpha_Blade_M, T_data_M=Talpha_Blade_Data_M, alpha_data_M=alpha_Blade_Data_M, BN_M=double(gcb)}
      mask prompts: TempDependence_M "TempDependence_M - Temperature dependence of the thermal expansion coefficient (unchecked - constant, checked - temperature dependent)"; alpha_M "alpha_M - Constant thermal expansion coefficient"; T_data_M "T_data_M - Temperature array (nx1)"; alpha_data_M "alpha_data_M - Thermal expansion coefficient array (nx1)"; BN_M "Block Name"
      mask help:
      | This function calculates the length or radius of a structure that has expanded or contracted due to thermal expansion. The block accepts the previous/reference length (Lo), previous/reference temperature (To), and current temperature (Tf) as its inputs. The user has the option to specify a constant thermal expansion coefficient or to incorporate temperature dependence by providing data that correlates the thermal expansion coefficient with temperature.
      |
      | This block is capable of accepting various units but it is important that the units be consistent across all inputs and parameters. For details on this block, see the block help menu.
      mask init:
      | %set default parameters if they are not being used
      | if TempDependence_M == 0
      |     T_data_M = [0 5000];
      |     alpha_data_M = [10e-6 10e-6];
      | elseif TempDependence_M == 1
      |     alpha_M = 10e-6;
      | end
      mask Help: web(which('Deformation_TSAT_ThermExp1DElastic.html'),'-helpbrowser')
      mask Callback TempDependence_M:
      | MSK_SEC_Enables_TSAT('TempDependence_M',2,'dis')
      | MSK_SEC_Enables_TSAT('TempDependence_M',[3 4],'en')
  Blade Length after Thermal Expansion : Outport
  wires:
  Average Rotor Temperature/1 -> Thermal Expansion 1D Elastic/3(Current Temperature [Tf]), Memory1/1
  Memory2/1 -> Thermal Expansion 1D Elastic/1(Previous/Reference Length [Lo])
  Memory1/1 -> Thermal Expansion 1D Elastic/2(Previous/Reference Temperature [To])
  Thermal Expansion 1D Elastic/1(Current Length [L]) -> Memory2/1, Blade Length after Thermal Expansion/1

== system lib_TCML/Dynamic Tip Clearance/Blade Deformation/Deformation1/Deformation Due To Centrifugal Forces ==
  Shaft Speed [N] (rpm) : Inport
  Average Temperature : Inport  Port=2
  Blade Length After Thermal Expansion : Inport  Port=3
  Rotor Outer Radius : Inport  Port=4
  Add : Sum
  Constant Young's Modulus : Constant  Value=E_Blade_M
  Density of Rotor : Constant  Value=rho_Blade_M
  Density of Rotor1 : Constant
  Divide : Product  Inputs=/*
  Divide1 : Product  Inputs=****
  Divide2 : Product  Inputs=**
  E Temperature Dependence? : Constant  Value=E_TempDependence_Blade_M
  Gain1 : Gain  Gain=2*pi/60
  Math Function : Math  Operator=square  SaturateOnIntegerOverflow=on
  Math Function2 : Math  Operator=square  SaturateOnIntegerOverflow=on
  Switch : Switch  Criteria=u2 > Threshold
  Young's Modulus vs. Temperature : Lookup_n-D  NumberOfTableDimensions=1  BreakpointsForDimension1=TE_Blade_Data_M  Table=E_Blade_Data_M  InternalRulePriority=Speed  RndMeth=Simplest  InputSameDT=on
  Blade Length : Outport
  wires:
  Divide2/1 -> Divide1/4
  Math Function2/1 -> Divide2/2
  Add/1 -> Divide2/1
  Rotor Outer Radius/1 -> Add/1
  Blade Length After Thermal Expansion/1 -> Math Function2/1, Add/2
  Average Temperature/1 -> Young's Modulus vs. Temperature/1
  Divide1/1 -> Blade Length/1
  Shaft Speed [N] (rpm)/1 -> Gain1/1
  Math Function/1 -> Divide1/2
  E Temperature Dependence?/1 -> Switch/2
  Density of Rotor/1 -> Divide1/3
  Gain1/1 -> Math Function/1  "rad/sec"
  Switch/1 -> Divide/1
  Divide/1 -> Divide1/1
  Constant Young's Modulus/1 -> Switch/3
  Density of Rotor1/1 -> Divide/2
  Young's Modulus vs. Temperature/1 -> Switch/1

== system lib_TCML/Dynamic Tip Clearance/Blade Deformation/Deformation1/Deformation Due To Thermal Expansion ==
  Average Blade Temperature : Inport
  Memory1 : Memory  X0=T0_Blade_M
  Memory2 : Memory  X0=L_Blade_M
  Thermal Expansion 1D Elastic : Subsystem  mask(TSAT: Thermal Expansion Library Block){TempDependence_M=on, alpha_M=alpha_Blade_M, T_data_M=Talpha_Blade_Data_M, alpha_data_M=alpha_Blade_Data_M, BN_M=double(gcb)}
      mask prompts: TempDependence_M "TempDependence_M - Temperature dependence of the thermal expansion coefficient (unchecked - constant, checked - temperature dependent)"; alpha_M "alpha_M - Constant thermal expansion coefficient"; T_data_M "T_data_M - Temperature array (nx1)"; alpha_data_M "alpha_data_M - Thermal expansion coefficient array (nx1)"; BN_M "Block Name"
      mask help:
      | This function calculates the length or radius of a structure that has expanded or contracted due to thermal expansion. The block accepts the previous/reference length (Lo), previous/reference temperature (To), and current temperature (Tf) as its inputs. The user has the option to specify a constant thermal expansion coefficient or to incorporate temperature dependence by providing data that correlates the thermal expansion coefficient with temperature.
      |
      | This block is capable of accepting various units but it is important that the units be consistent across all inputs and parameters. For details on this block, see the block help menu.
      mask init:
      | %set default parameters if they are not being used
      | if TempDependence_M == 0
      |     T_data_M = [0 5000];
      |     alpha_data_M = [10e-6 10e-6];
      | elseif TempDependence_M == 1
      |     alpha_M = 10e-6;
      | end
      mask Help: web(which('Deformation_TSAT_ThermExp1DElastic.html'),'-helpbrowser')
      mask Callback TempDependence_M:
      | MSK_SEC_Enables_TSAT('TempDependence_M',2,'dis')
      | MSK_SEC_Enables_TSAT('TempDependence_M',[3 4],'en')
  Blade Length after Thermal Expansion : Outport
  wires:
  Thermal Expansion 1D Elastic/1(Current Length [L]) -> Blade Length after Thermal Expansion/1, Memory2/1
  Memory1/1 -> Thermal Expansion 1D Elastic/2(Previous/Reference Temperature [To])
  Memory2/1 -> Thermal Expansion 1D Elastic/1(Previous/Reference Length [Lo])
  Average Blade Temperature/1 -> Memory1/1, Thermal Expansion 1D Elastic/3(Current Temperature [Tf])

== system lib_TCML/Dynamic Tip Clearance/Case Deformation/Deformation/Thermal Expansion 1D Elastic ==
  Previous/Reference Length [Lo] : Inport
  Previous/Reference Temperature [To] : Inport  Port=2
  Current Temperature [Tf] : Inport  Port=3
  Add : Sum  Inputs=+-
  Add1 : Sum
  MATLAB Function : MATLAB Function  TreatAsAtomicUnit=on
  Mass Flow Rate on Inner Surface1 : Constant  Value=TempDependence_M
  Mass Flow Rate on Inner Surface2 : Constant  Value=T_data_M
  Mass Flow Rate on Inner Surface3 : Constant  Value=alpha_data_M
  Mass Flow Rate on Inner Surface4 : Constant  Value=alpha_M
  Mass Flow Rate on Inner Surface6 : Constant  Value=BN_M
  Memory : Memory  X0=zeros(1,7)  InheritSampleTime=on
  Product : Product  Inputs=***
  Switch : Switch  Criteria=u2 > Threshold
  Current Length [L] : Outport
  wires:
  Previous/Reference Length [Lo]/1 -> Product/2, Add1/2, MATLAB Function/3(Lo)
  Previous/Reference Temperature [To]/1 -> MATLAB Function/4(To), Add/2
  Current Temperature [Tf]/1 -> MATLAB Function/5(Tf), Add/1
  Mass Flow Rate on Inner Surface6/1 -> MATLAB Function/7(BN)
  MATLAB Function/1(L) -> Switch/1
  Memory/1 -> MATLAB Function/6(Erro)
  MATLAB Function/2(Err) -> Memory/1
  Mass Flow Rate on Inner Surface1/1 -> Switch/2
  Mass Flow Rate on Inner Surface2/1 -> MATLAB Function/1(T_data)
  Mass Flow Rate on Inner Surface3/1 -> MATLAB Function/2(alpha_data)
  Add/1 -> Product/1
  Mass Flow Rate on Inner Surface4/1 -> Product/3
  Switch/1 -> Current Length [L]/1
  Product/1 -> Add1/1
  Add1/1 -> Switch/3
